simulink model "first_controller"  (R2020a)
settings: Solver=VariableStepAuto  StartTime=0.0  StopTime=10.0  RelTol=1e-3
libraries: vrlib x1, simulink x1
settings Model: Creator=angelo  LastModifiedBy=angelo

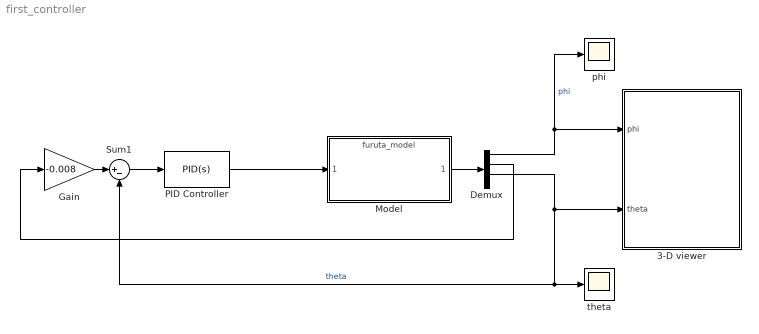
== system first_controller ==
  3-D viewer : Subsystem
  Demux : Demux
  Gain : Gain  Gain=-0.008
  Model : ModelReference  ModelNameDialog=furuta_model.slx  SimulationMode=Normal  ModelReferenceVersion=1.21
  PID Controller : simulink/Continuous/PID Controller  Controller=PID  Form=Parallel  TimeDomain=Continuous-time  UseExternalTs=off  SampleTime=-1  IntegratorMethod=Forward Euler  FilterMethod=Forward Euler  ControllerParametersSource=internal  P=-18  I=-25  D=-2.5  UseFilter=on  N=10  TunerSelectOption=Transfer Function Based (PID Tuner App)  InitialConditionSource=internal  InitialConditionForIntegrator=0  InitialConditionForFilter=0  DifferentiatorICPrevScaledInput=0  ExternalReset=none  TrackingMode=off  Kt=1  LimitOutput=on  UpperSaturationLimit=10  LowerSaturationLimit=-10  LinearizeAsGain=on  AntiWindupMode=clamping  Kb=1  POutMin=[]  POutMax=[]  IOutMin=[]  IOutMax=[]  DOutMin=[]  DOutMax=[]  NOutMin=[]  NOutMax=[]  SumOutMin=[]  SumOutMax=[]  SaturationOutMin=[]  SaturationOutMax=[]  PParamMin=[]  PParamMax=[]  IParamMin=[]  IParamMax=[]  DParamMin=[]  DParamMax=[]  NParamMin=[]  NParamMax=[]  KbParamMin=[]  KbParamMax=[]  KtParamMin=[]  KtParamMax=[]  KbOutMin=[]  KbOutMax=[]  KtOutMin=[]  KtOutMax=[]  IntegratorOutMin=[]  IntegratorOutMax=[]  FilterOutMin=[]  FilterOutMax=[]  SumI1OutMin=[]  SumI1OutMax=[]  SumI2OutMin=[]  SumI2OutMax=[]  SumI3OutMin=[]  SumI3OutMax=[]  SumI4OutMin=[]  SumI4OutMax=[]  SumDOutMin=[]  SumDOutMax=[]  DifferentiatorOutMin=[]  DifferentiatorOutMax=[]  FilterDiffOutCoefMin=[]  FilterDiffOutCoefMax=[]  ReciprocalOutMin=[]  ReciprocalOutMax=[]  SumDenOutMin=[]  SumDenOutMax=[]  SumNumOutMin=[]  SumNumOutMax=[]  DivideOutMin=[]  DivideOutMax=[]  UdiffTsProdOutMin=[]  UdiffTsProdOutMax=[]  NTsProdOutMin=[]  NTsProdOutMax=[]  UintegralTsProdOutMin=[]  UintegralTsProdOutMax=[]  UngainTsProdOutMin=[]  UngainTsProdOutMax=[]  IntegratorContinuousStateAttributes=''  IntegratorStateMustResolveToSignalObject=off  IntegratorRTWStateStorageClass=Auto  FilterContinuousStateAttributes=''  FilterStateMustResolveToSignalObject=off  FilterRTWStateStorageClass=Auto  ParallelPVariant=InternalParameters  IdealPVariant=Disabled  IVariant=InternalParameters  DVariant=InternalParameters  IntegratorVariant=Continuous  SatVariant=Enabled  AWVariant=ContClampingParallel  PCopyVariant=Disabled  TRVariant=Disabled  FdbkBlocksVariant=Forward  IdealPFdbkVariant=Disabled  SatFdbkVariant=Disabled  DerivativeFilterVariant=ContFilter  NVariant=InternalParameters  NCopyVariant=Disabled  FilterICVariant=InternalICsFilter  IntegratorICVariant=InternalICs  ExternalResetVariant=Disabled  TRSumVariant=Passthrough  SumFdbkVariant=Disabled  SumVariant=Sum_PID  TsampFilterVariant=InternalTs  TsampNgainVariant=Passthrough  TsampIntegralVariant=Passthrough
  Sum1 : Sum  Inputs=|+-
  phi : Scope
  theta : Scope
  wires:
  Sum1/1 -> PID Controller/1
  Demux/1 -> phi/1, 3-D viewer/1(phi)  "phi"
  Gain/1 -> Sum1/1
  Demux/3 -> Sum1/2, theta/1, 3-D viewer/2(theta)  "theta"
  Model/1 -> Demux/1
  PID Controller/1 -> Model/1
  Demux/2 -> Gain/1

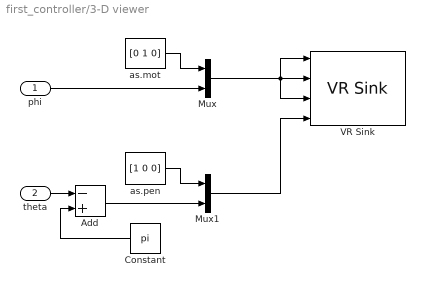
== system first_controller/3-D viewer ==
  phi : Inport
  theta : Inport  Port=2
  Add : Sum  Inputs=-+
  Constant : Constant  Value=pi
  Mux : Mux  Inputs=2
  Mux1 : Mux  Inputs=2
  VR Sink : vrlib/VR Sink  InstantiateOnLoad=on  SampleTime=0.04  ViewEnable=on  RemoteChange=off  RemoteView=on  FieldsWritten=Puleggia_8.rotation.4.1.1.double#Puleggia.rotation.4.1.1.double#LinkP-L.rotation.4.1.1.double#pispolo.rotation.4.1.1.double  WorldFileName=fu.wrl  AutoView=off  VideoDimensions=[]  AllowVariableSize=off
  as.mot : Constant  Value=[0 1 0]
  as.pen : Constant  Value=[1 0 0]
  wires:
  as.mot/1 -> Mux/1
  as.pen/1 -> Mux1/1
  Mux/1 -> VR Sink/1, VR Sink/3, VR Sink/2
  Mux1/1 -> VR Sink/4
  Add/1 -> Mux1/2
  Constant/1 -> Add/2
  phi/1 -> Mux/2
  theta/1 -> Add/1
